simulink model "simulinkModel"  (R2024a)
settings: Solver=VariableStepAuto  StartTime=0.0  StopTime=10.0  RelTol=1e-3
values from neighbouring files (symbols this model uses):
  G_h = 3600*3000    (= 10800000)    [control.m]
  K1 = 1/4.285e-7    (= 2333722.28705)    [control.m]
  K2 = 1/(1470*1005.4)    (= 6.76618369647e-07)    [control.m]
  Kd = 0.012    [control.m]
  Ki = 5.5    [control.m]
  Kp = 0.01    [control.m]
  setTemp = 5    [control.m]
  T_heater = 70    [control.m]
  Ts = 0.1    [control.m]
libraries: simulink x1, slpidlib x1
settings Model: Creator=mnepr  LastModifiedBy=mnepr

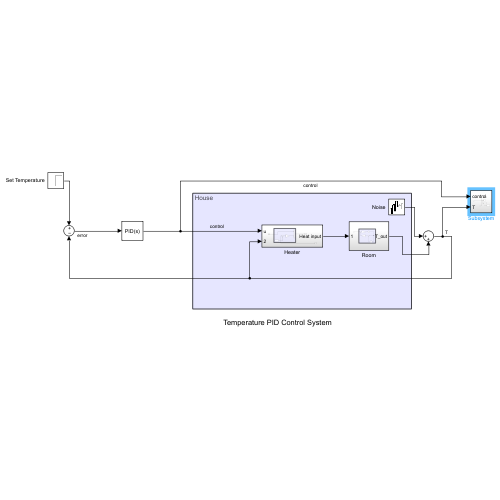
[thumbnail: Simulink's stored preview of the top-level diagram]
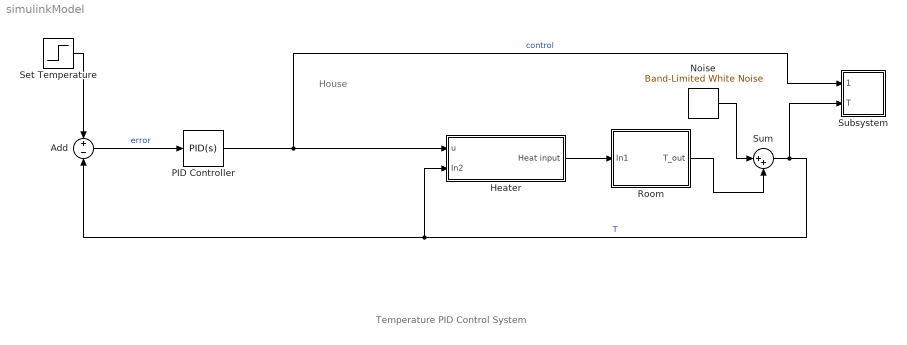
== system simulinkModel ==
  note: House
  note: Temperature PID Control System
  Add : Sum  Inputs=+-
  Heater : Subsystem
  Noise : simulink/Sources/Band-Limited White Noise  Cov=Np  Ts=Ts  seed=[23341]
  PID Controller : slpidlib/PID Controller  Controller=PID  Form=Parallel  TimeDomain=Continuous-time  UseExternalTs=off  SampleTime=-1  IntegratorMethod=Forward Euler  FilterMethod=Forward Euler  ControllerParametersSource=internal  P=Kp  I=Ki  UseKiTs=off  D=Kd  UseExternalDerivativeSource=off  N=100  UseFilter=on  TunerSelectOption=Transfer Function Based (PID Tuner App)  InitialConditionSource=internal  InitialConditionForIntegrator=0  InitialConditionForFilter=0  DifferentiatorICPrevScaledInput=0  ExternalReset=none  TrackingMode=off  Kt=1  LimitOutput=off  SatLimitsSource=internal  UpperSaturationLimit=inf  LowerSaturationLimit=-inf  LinearizeAsGain=on  AntiWindupMode=none  Kb=1  LimitIntegrator=off  UpperIntegratorSaturationLimit=inf  LowerIntegratorSaturationLimit=-inf  POutMin=[]  POutMax=[]  IOutMin=[]  IOutMax=[]  DOutMin=[]  DOutMax=[]  NOutMin=[]  NOutMax=[]  SumOutMin=[]  SumOutMax=[]  SaturationOutMin=[]  SaturationOutMax=[]  PParamMin=[]  PParamMax=[]  IParamMin=[]  IParamMax=[]  DParamMin=[]  DParamMax=[]  NParamMin=[]  NParamMax=[]  KbParamMin=[]  KbParamMax=[]  KtParamMin=[]  KtParamMax=[]  KbOutMin=[]  KbOutMax=[]  KtOutMin=[]  KtOutMax=[]  IntegratorOutMin=[]  IntegratorOutMax=[]  FilterOutMin=[]  FilterOutMax=[]  SumI1OutMin=[]  SumI1OutMax=[]  SumI2OutMin=[]  SumI2OutMax=[]  SumI3OutMin=[]  SumI3OutMax=[]  SumI4OutMin=[]  SumI4OutMax=[]  SumDOutMin=[]  SumDOutMax=[]  DifferentiatorOutMin=[]  DifferentiatorOutMax=[]  FilterDiffOutCoefMin=[]  FilterDiffOutCoefMax=[]  ReciprocalOutMin=[]  ReciprocalOutMax=[]  SumDenOutMin=[]  SumDenOutMax=[]  SumNumOutMin=[]  SumNumOutMax=[]  DivideOutMin=[]  DivideOutMax=[]  UdiffTsProdOutMin=[]  UdiffTsProdOutMax=[]  NTsProdOutMin=[]  NTsProdOutMax=[]  UintegralTsProdOutMin=[]  UintegralTsProdOutMax=[]  UngainTsProdOutMin=[]  UngainTsProdOutMax=[]  ClampingZeroOutDataTypeStr=Inherit: Inherit via back propagation  ClampingZeroOutMin=[]  ClampingZeroOutMax=[]  FilterDenConstantOutDataTypeStr=Inherit: Inherit via back propagation  FilterDenConstantOutMin=[]  FilterDenConstantOutMax=[]  PCopyOutDataTypeStr=Inherit: Inherit via back propagation  PCopyOutMin=[]  PCopyOutMax=[]  NCopyOutDataTypeStr=Inherit: Inherit via back propagation  NCopyOutMin=[]  NCopyOutMax=[]  IntegratorContinuousStateAttributes=''  IntegratorStateMustResolveToSignalObject=off  IntegratorRTWStateStorageClass=Auto  FilterContinuousStateAttributes=''  FilterStateMustResolveToSignalObject=off  FilterRTWStateStorageClass=Auto  ParallelPVariant=InternalParameters  IdealPVariant=Disabled  IVariant=InternalParameters  DVariant=InternalParameters  IntegratorVariant=Continuous  SatVariant=Disabled  AWVariant=Passthrough  PCopyVariant=Disabled  TRVariant=Disabled  FdbkBlocksVariant=Forward  IdealPFdbkVariant=Disabled  SatFdbkVariant=Disabled  DerivativeFilterVariant=ContFilter  NVariant=InternalParameters  NCopyVariant=Disabled  FilterICVariant=InternalICsFilter  IntegratorICVariant=InternalICs  ExternalResetVariant=Disabled  TRSumVariant=Passthrough  SumFdbkVariant=Disabled  SumVariant=Sum_PID  TsampFilterVariant=InternalTs  TsampNgainVariant=Passthrough  TsampIntegralVariant=Passthrough  ExternalSaturationOutDataTypeStr=Inherit: Same as second input  DerivativeSourceVariant=ErrorSignal
  Room : Subsystem
  Set Temperature : Step  After=setTemp  SampleTime=0
  Subsystem : Subsystem
  Sum : Sum  Inputs=|++
  wires:
  PID Controller/1 -> Subsystem/1(control), Heater/1(u)  "control"
  Heater/1(Heat input) -> Room/1(In1)
  Add/1 -> PID Controller/1  "error"
  Noise/1 -> Sum/1
  Room/1(T_out) -> Sum/2
  Sum/1 -> Subsystem/2(T), Heater/2(In2), Add/2  "T"
  Set Temperature/1 -> Add/1

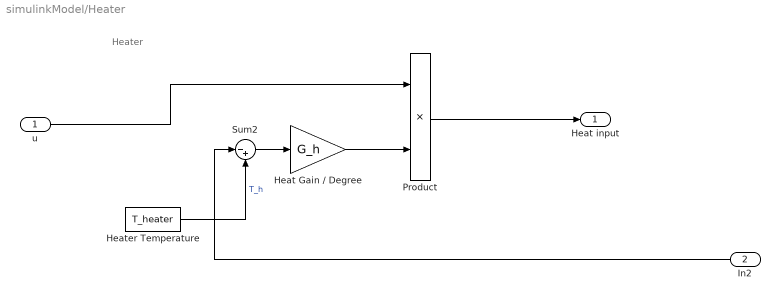
== system simulinkModel/Heater ==
  note: Heater
  u : Inport
  In2 : Inport  Port=2
  Heat Gain / Degree : Gain  Gain=G_h
  Heater Temperature : Constant  Value=T_heater  VectorParams1D=off
  Product : Product  RndMeth=Zero
  Sum2 : Sum  Inputs=|-+
  Heat input : Outport
  wires:
  In2/1 -> Sum2/1
  Heater Temperature/1 -> Sum2/2  "T_h"
  Sum2/1 -> Heat Gain / Degree/1
  Heat Gain / Degree/1 -> Product/2
  Product/1 -> Heat input/1
  u/1 -> Product/1

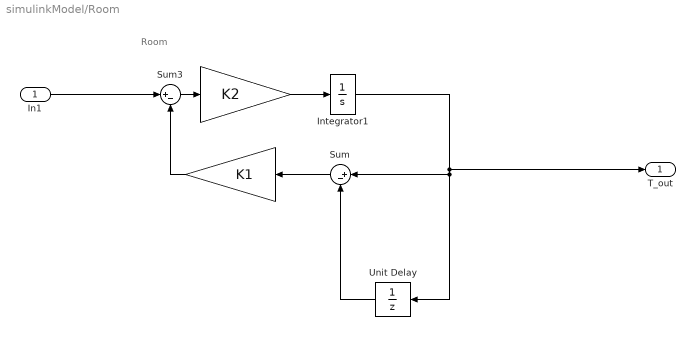
== system simulinkModel/Room ==
  note: Room
  In1 : Inport
  " " : Gain  Gain=K1  SaturateOnIntegerOverflow=on  OutDataTypeStr=Inherit: Same as input  ParamDataTypeStr=Inherit: Same as input
  "  " : Gain  Gain=K2  SaturateOnIntegerOverflow=on  OutDataTypeStr=Inherit: Same as input  ParamDataTypeStr=Inherit: Same as input
  Integrator1 : Integrator
  Sum : Sum  Inputs=|+-
  Sum3 : Sum  Inputs=|+-  InputSameDT=on  SaturateOnIntegerOverflow=on  OutDataTypeStr=Inherit: Same as first input
  Unit Delay : UnitDelay  SampleTime=0.001  HasFrameUpgradeWarning=on
  T_out : Outport
  wires:
  In1/1 -> Sum3/1
  Unit Delay/1 -> Sum/2
  Integrator1/1 -> Unit Delay/1, Sum/1, T_out/1
  " "/1 -> Sum3/2
  "  "/1 -> Integrator1/1
  Sum3/1 -> "  "/1
  Sum/1 -> " "/1

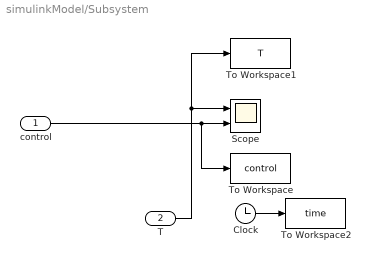
== system simulinkModel/Subsystem ==
  control : Inport
  T : Inport  Port=2
  Clock : Clock
  Scope : Scope  NumInputPorts=2
  To Workspace : ToWorkspace  VariableName=control
      settings: Save2DSignal=2-D array (concatenate along first dimension)
  To Workspace1 : ToWorkspace  VariableName=T
      settings: Save2DSignal=2-D array (concatenate along first dimension)
  To Workspace2 : ToWorkspace  VariableName=time
      settings: Save2DSignal=2-D array (concatenate along first dimension)
  wires:
  T/1 -> To Workspace1/1, Scope/1
  control/1 -> To Workspace/1, Scope/2
  Clock/1 -> To Workspace2/1
